simulink model "Simulink_asserv_Disc_10Avril_V2023a"  (R2023a)
settings: Solver=ode45  StartTime=0.0  StopTime=2500  FixedStep=0.01  RelTol=1e-3
undefined symbols (not defined in the file): AmbiantTemp, CondSig_mesureTemp_Gain, CondSig_mesureTemp_Vsub, Consigne1_Temps, Consigne1_Valeur, Consigne2_Temps, Consigne2_Valeur, Consigne3_Temps, Consigne3_Valeur, DivTen_mesureTemp_R_pullup, DivTen_mesureTemp_Vcc, Gain_Comparateur_VoltageControle, GuT1_Denominateur, GuT1_Numerateur, GuT2_Denominateur, GuT2_Numerateur, GuT3_Denominateur, GuT3_Numerateur, NbrsBits_ADC, NbrsBits_DAC, Perturbation_Resistance, Perturbation_TempsApplication, Perturbation_Tension, PerturbT1_Denominateur, PerturbT1_Numerateur, PerturbT2_Denominateur, PerturbT2_Numerateur, PerturbT3_Denominateur, PerturbT3_Numerateur, RC_deno, Regulateur_Denominateur, Regulateur_Numerateur, SaturationLimite_inferieure, SaturationLimite_superieure, setupDelay, SourceCourant_Gain_Vcontrole_vers_A, T1T3_Denominateur, T1T3_Numerateur, T2T3_Denominateur, T2T3_Numerateur, ThermoRes_SH_A, ThermoRes_SH_B, ThermoRes_SH_C, ThermoRes_SH_D, ThermoRes_SH_R_nom, ThermoRes_SHTEMP_A, ThermoRes_SHTEMP_B, ThermoRes_SHTEMP_C, ThermoRes_SHTEMP_D
libraries: simulink x2
settings Model: Creator=alcot161  LastModifiedBy=alcot161
settings RTWCC: GPUComputeCapability=5.0

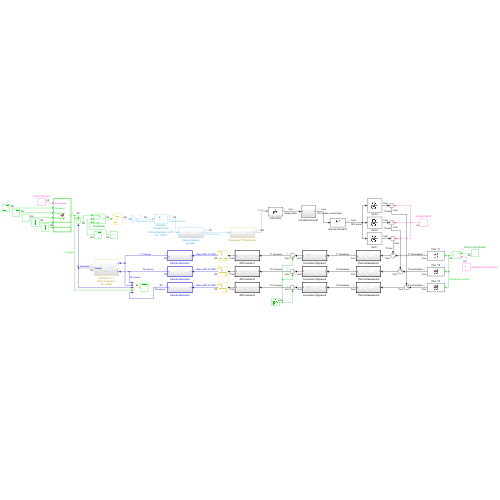
[thumbnail: Simulink's stored preview of the top-level diagram]
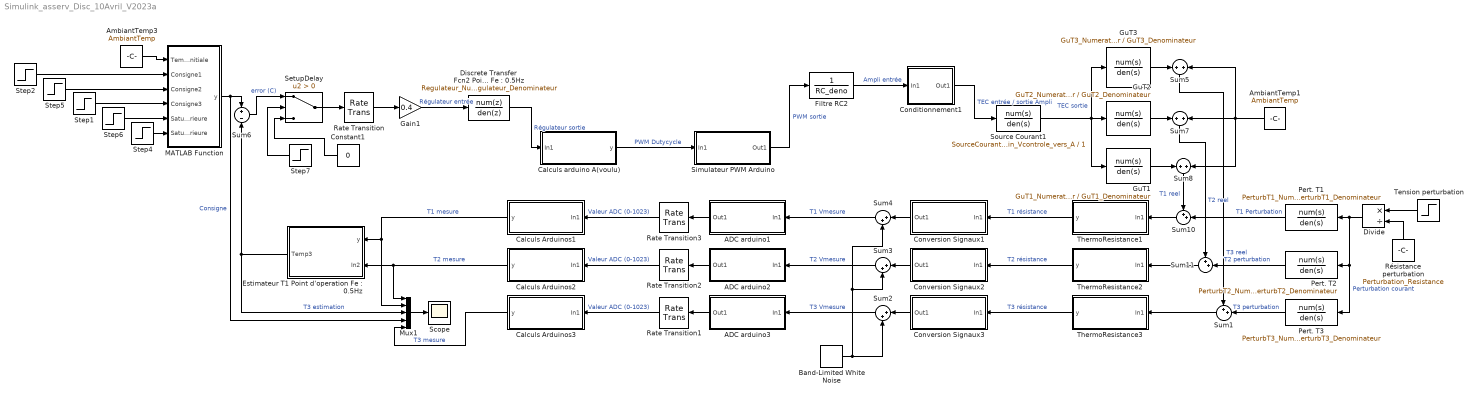
== system Simulink_asserv_Disc_10Avril_V2023a ==
  ADC arduino1 : Subsystem  TreatAsAtomicUnit=on
  ADC arduino2 : Subsystem  TreatAsAtomicUnit=on
  ADC arduino3 : Subsystem  TreatAsAtomicUnit=on
  AmbiantTemp1 : Constant  Value=AmbiantTemp
  AmbiantTemp3 : Constant  Value=AmbiantTemp
  Band-Limited White Noise : simulink/Sources/Band-Limited White Noise  Cov=BruitMesure  Ts=0.05  seed=[23341]
  Calculs Arduinos1 : Subsystem  TreatAsAtomicUnit=on
  Calculs Arduinos2 : Subsystem  TreatAsAtomicUnit=on
  Calculs Arduinos3 : Subsystem  TreatAsAtomicUnit=on
  "Calculs arduino A(voulu) " : Subsystem
  Conditionnement1 : Subsystem
  Constant1 : Constant  Value=0  SampleTime=0.05
  Conversion Signaux1 : Subsystem  TreatAsAtomicUnit=on
  Conversion Signaux2 : Subsystem  TreatAsAtomicUnit=on
  Conversion Signaux3 : Subsystem  TreatAsAtomicUnit=on
  "Discrete Transfer Fcn2 Point d'operation : 27C Fe : 0.5Hz" : DiscreteTransferFcn  Numerator=Regulateur_Numerateur  Denominator=Regulateur_Denominateur
  Divide : Product  Inputs=*/
  "Estimateur T1 Point d'operation Fe : 0.5Hz" : Subsystem
  Filtre RC2 : TransferFcn  Denominator=RC_deno
  Gain1 : Gain  Gain=0.4
  GuT1 : TransferFcn  Numerator=GuT1_Numerateur  Denominator=GuT1_Denominateur
  GuT2 : TransferFcn  Numerator=GuT2_Numerateur  Denominator=GuT2_Denominateur
  GuT3 : TransferFcn  Numerator=GuT3_Numerateur  Denominator=GuT3_Denominateur
  MATLAB Function : MATLAB Function  TreatAsAtomicUnit=on
  Mux1 : Mux  Inputs=5
  Pert. T1 : TransferFcn  Numerator=PerturbT1_Numerateur  Denominator=PerturbT1_Denominateur
  Pert. T2 : TransferFcn  Numerator=PerturbT2_Numerateur  Denominator=PerturbT2_Denominateur
  Pert. T3 : TransferFcn  Numerator=PerturbT3_Numerateur  Denominator=PerturbT3_Denominateur
  Rate Transition : RateTransition  OutPortSampleTime=PeriodEchant_asserv
  Rate Transition1 : RateTransition  OutPortSampleTime=PeriodeEchant_temp
  Rate Transition2 : RateTransition  OutPortSampleTime=PeriodeEchant_temp
  Rate Transition3 : RateTransition  OutPortSampleTime=PeriodeEchant_temp
  Résistance perturbation : Constant  Value=Perturbation_Resistance
  Scope : Scope
  SetupDelay : Switch  Criteria=u2 > Threshold  SaturateOnIntegerOverflow=off  InputSameDT=off
  Simulateur PWM Arduino : Subsystem
  Source Courant1 : TransferFcn  Numerator=SourceCourant_Gain_Vcontrole_vers_A  Denominator=1
  Step1 : Step  Time=Consigne3_Temps  After=Consigne3_Valeur  SampleTime=0.05
  Step2 : Step  Time=Consigne1_Temps  After=Consigne1_Valeur  SampleTime=0.05
  Step4 : Step  Time=0  After=SaturationLimite_inferieure  SampleTime=0.05
  Step5 : Step  Time=Consigne2_Temps  After=Consigne2_Valeur  SampleTime=0.05
  Step6 : Step  Time=0  After=SaturationLimite_superieure  SampleTime=0.05
  Step7 : Step  Time=setupDelay  SampleTime=0.05
  Sum1 : Sum  Inputs=++|
  Sum10 : Sum  Inputs=++|
  Sum11 : Sum  Inputs=++|
  Sum2 : Sum  Inputs=|++
  Sum3 : Sum  Inputs=|++
  Sum4 : Sum  Inputs=|++
  Sum5 : Sum  Inputs=+|+
  Sum6 : Sum  Inputs=+|-
  Sum7 : Sum  Inputs=+|+
  Sum8 : Sum  Inputs=+|+
  Tension perturbation : Step  Time=Perturbation_TempsApplication  After=Perturbation_Tension  SampleTime=0.05
  ThermoResistance1 : Subsystem  TreatAsAtomicUnit=on
  ThermoResistance2 : Subsystem  TreatAsAtomicUnit=on
  ThermoResistance3 : Subsystem  TreatAsAtomicUnit=on
  wires:
  ThermoResistance2/1(y) -> Conversion Signaux2/1(In1)  "T2 résistance"
  GuT2/1 -> Sum7/1
  Conversion Signaux2/1(Out1) -> Sum3/1
  Rate Transition2/1 -> Calculs Arduinos2/1(In1)  "Valeur ADC (0-1023)"
  Simulateur PWM Arduino/1(Out1) -> Filtre RC2/1  "PWM sortie"
  Step5/1 -> MATLAB Function/3(Consigne2)
  Conversion Signaux1/1(Out1) -> Sum4/1
  AmbiantTemp1/1 -> Sum5/2, Sum8/2, Sum7/2
  Filtre RC2/1 -> Conditionnement1/1(In1)  "Ampli entrée"
  Calculs Arduinos1/1(y) -> Mux1/2, "Estimateur T1 Point d'operation Fe : 0.5Hz"/1(y)  "T1 mesure"
  Rate Transition3/1 -> Calculs Arduinos1/1(In1)  "Valeur ADC (0-1023)"
  "Calculs arduino A(voulu) "/1(y) -> Simulateur PWM Arduino/1(In1)  "PWM Dutycycle"
  Calculs Arduinos2/1(y) -> "Estimateur T1 Point d'operation Fe : 0.5Hz"/2(In2), Mux1/1  "T2 mesure"
  Source Courant1/1 -> GuT3/1, GuT1/1, GuT2/1  "TEC sortie"
  ThermoResistance1/1(y) -> Conversion Signaux1/1(In1)  "T1 résistance"
  Sum7/1 -> Sum11/1  "T2 reel"
  Conditionnement1/1(Out1) -> Source Courant1/1  "TEC entrée / sortie Ampli"
  GuT1/1 -> Sum8/1
  GuT3/1 -> Sum5/1
  "Discrete Transfer Fcn2 Point d'operation : 27C Fe : 0.5Hz"/1 -> "Calculs arduino A(voulu) "/1(In1)  "Régulateur sortie"
  "Estimateur T1 Point d'operation Fe : 0.5Hz"/1(Temp3) -> Sum6/2, Mux1/3  "T3 estimation"
  Gain1/1 -> "Discrete Transfer Fcn2 Point d'operation : 27C Fe : 0.5Hz"/1  "Régulateur entrée"
  Sum6/1 -> SetupDelay/1  "error (C)"
  SetupDelay/1 -> Rate Transition/1
  Sum8/1 -> Sum10/1  "T1 reel"
  Sum10/1 -> ThermoResistance1/1(In1)
  Sum11/1 -> ThermoResistance2/1(In1)
  Step1/1 -> MATLAB Function/4(Consigne3)
  Résistance perturbation/1 -> Divide/2
  Tension perturbation/1 -> Divide/1
  Divide/1 -> Pert. T3/1, Pert. T2/1, Pert. T1/1  "Perturbation courant"
  Pert. T1/1 -> Sum10/2  "T1 Perturbation"
  AmbiantTemp3/1 -> MATLAB Function/1(TempInitiale)
  Step2/1 -> MATLAB Function/2(Consigne1)
  MATLAB Function/1(y) -> Mux1/4, Sum6/1  "Consigne"
  Calculs Arduinos3/1(y) -> Mux1/5  "T3 mesure"
  ThermoResistance3/1(y) -> Conversion Signaux3/1(In1)  "T3 résistance"
  Rate Transition1/1 -> Calculs Arduinos3/1(In1)  "Valeur ADC (0-1023)"
  Conversion Signaux3/1(Out1) -> Sum2/1
  Sum5/1 -> Sum1/1  "T3 reel"
  Pert. T2/1 -> Sum11/2  "T2 perturbation"
  Pert. T3/1 -> Sum1/2  "T3 perturbation"
  Sum1/1 -> ThermoResistance3/1(In1)
  Step4/1 -> MATLAB Function/6(SaturationLimiteInferieure)
  Step6/1 -> MATLAB Function/5(SaturationLimiteSuperieure)
  Constant1/1 -> SetupDelay/3
  Step7/1 -> SetupDelay/2
  Mux1/1 -> Scope/1
  Sum2/1 -> ADC arduino3/1(In1)  "T3 Vmesure"
  Sum3/1 -> ADC arduino2/1(In1)  "T2 Vmesure"
  Sum4/1 -> ADC arduino1/1(In1)  "T1 Vmesure"
  Band-Limited White Noise/1 -> Sum2/2, Sum4/2, Sum3/2
  ADC arduino3/1(Out1) -> Rate Transition1/1
  ADC arduino1/1(Out1) -> Rate Transition3/1
  ADC arduino2/1(Out1) -> Rate Transition2/1
  Rate Transition/1 -> Gain1/1

== system Simulink_asserv_Disc_10Avril_V2023a/ADC arduino1 ==
  In1 : Inport
  Floor : Rounding
  Gain2 : Gain  Gain=2^NbrsBits_ADC/5
  Out1 : Outport
  wires:
  In1/1 -> Gain2/1
  Gain2/1 -> Floor/1
  Floor/1 -> Out1/1

== system Simulink_asserv_Disc_10Avril_V2023a/ADC arduino2 ==
  In1 : Inport
  Floor : Rounding
  Gain2 : Gain  Gain=2^NbrsBits_ADC/5
  Out1 : Outport
  wires:
  Floor/1 -> Out1/1
  In1/1 -> Gain2/1
  Gain2/1 -> Floor/1

== system Simulink_asserv_Disc_10Avril_V2023a/ADC arduino3 ==
  In1 : Inport
  Floor : Rounding
  Gain2 : Gain  Gain=2^NbrsBits_ADC/5
  Out1 : Outport
  wires:
  Floor/1 -> Out1/1
  In1/1 -> Gain2/1
  Gain2/1 -> Floor/1

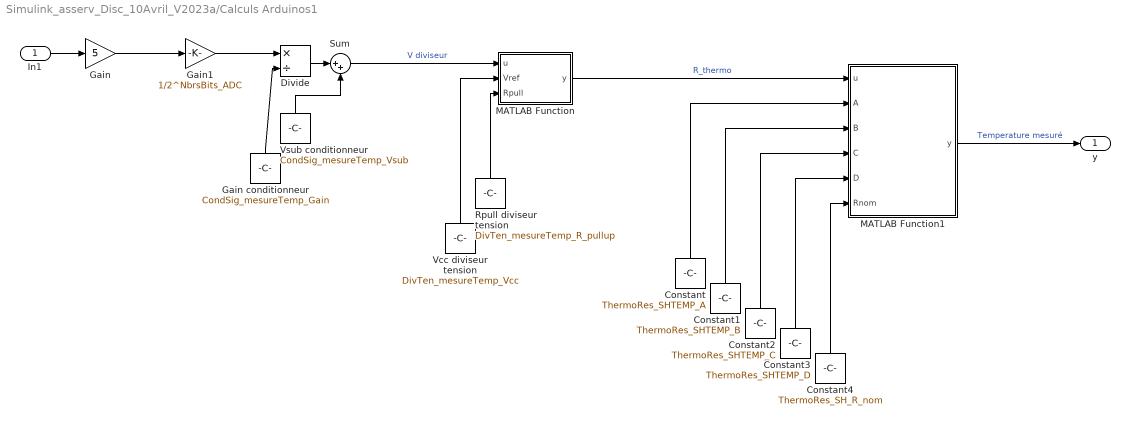
== system Simulink_asserv_Disc_10Avril_V2023a/Calculs Arduinos1 ==
  In1 : Inport
  Constant : Constant  Value=ThermoRes_SHTEMP_A
  Constant1 : Constant  Value=ThermoRes_SHTEMP_B
  Constant2 : Constant  Value=ThermoRes_SHTEMP_C
  Constant3 : Constant  Value=ThermoRes_SHTEMP_D
  Constant4 : Constant  Value=ThermoRes_SH_R_nom
  Divide : Product  Inputs=*/
  Gain : Gain  Gain=5
  Gain conditionneur : Constant  Value=CondSig_mesureTemp_Gain
  Gain1 : Gain  Gain=1/2^NbrsBits_ADC
  MATLAB Function : MATLAB Function  TreatAsAtomicUnit=on
  MATLAB Function1 : MATLAB Function  TreatAsAtomicUnit=on
  Rpull diviseur tension : Constant  Value=DivTen_mesureTemp_R_pullup
  Sum : Sum  Inputs=|++
  Vcc diviseur tension : Constant  Value=DivTen_mesureTemp_Vcc
  Vsub conditionneur : Constant  Value=CondSig_mesureTemp_Vsub
  y : Outport
  wires:
  In1/1 -> Gain/1
  Gain/1 -> Gain1/1
  Gain conditionneur/1 -> Divide/2
  Divide/1 -> Sum/1
  Vsub conditionneur/1 -> Sum/2
  Sum/1 -> MATLAB Function/1(u)  "V diviseur"
  Rpull diviseur tension/1 -> MATLAB Function/3(Rpull)
  Vcc diviseur tension/1 -> MATLAB Function/2(Vref)
  MATLAB Function/1(y) -> MATLAB Function1/1(u)  "R_thermo"
  Constant/1 -> MATLAB Function1/2(A)
  Constant1/1 -> MATLAB Function1/3(B)
  Constant2/1 -> MATLAB Function1/4(C)
  Constant3/1 -> MATLAB Function1/5(D)
  Constant4/1 -> MATLAB Function1/6(Rnom)
  MATLAB Function1/1(y) -> y/1  "Temperature mesuré"
  Gain1/1 -> Divide/1

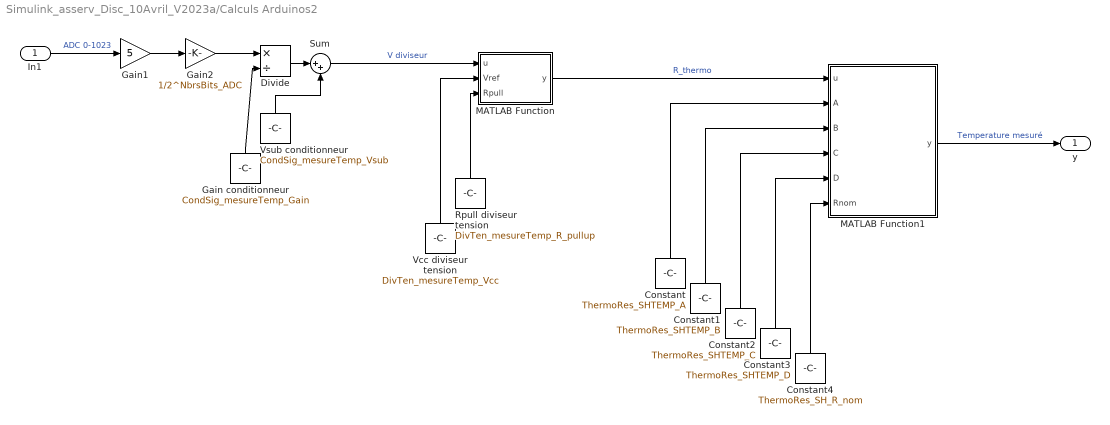
== system Simulink_asserv_Disc_10Avril_V2023a/Calculs Arduinos2 ==
  In1 : Inport
  Constant : Constant  Value=ThermoRes_SHTEMP_A
  Constant1 : Constant  Value=ThermoRes_SHTEMP_B
  Constant2 : Constant  Value=ThermoRes_SHTEMP_C
  Constant3 : Constant  Value=ThermoRes_SHTEMP_D
  Constant4 : Constant  Value=ThermoRes_SH_R_nom
  Divide : Product  Inputs=*/
  Gain conditionneur : Constant  Value=CondSig_mesureTemp_Gain
  Gain1 : Gain  Gain=5
  Gain2 : Gain  Gain=1/2^NbrsBits_ADC
  MATLAB Function : MATLAB Function  TreatAsAtomicUnit=on
  MATLAB Function1 : MATLAB Function  TreatAsAtomicUnit=on
  Rpull diviseur tension : Constant  Value=DivTen_mesureTemp_R_pullup
  Sum : Sum  Inputs=|++
  Vcc diviseur tension : Constant  Value=DivTen_mesureTemp_Vcc
  Vsub conditionneur : Constant  Value=CondSig_mesureTemp_Vsub
  y : Outport
  wires:
  Gain conditionneur/1 -> Divide/2
  Divide/1 -> Sum/1
  Vsub conditionneur/1 -> Sum/2
  Sum/1 -> MATLAB Function/1(u)  "V diviseur"
  Rpull diviseur tension/1 -> MATLAB Function/3(Rpull)
  Vcc diviseur tension/1 -> MATLAB Function/2(Vref)
  MATLAB Function/1(y) -> MATLAB Function1/1(u)  "R_thermo"
  Constant/1 -> MATLAB Function1/2(A)
  Constant1/1 -> MATLAB Function1/3(B)
  Constant2/1 -> MATLAB Function1/4(C)
  Constant3/1 -> MATLAB Function1/5(D)
  Constant4/1 -> MATLAB Function1/6(Rnom)
  MATLAB Function1/1(y) -> y/1  "Temperature mesuré"
  Gain2/1 -> Divide/1
  In1/1 -> Gain1/1  "ADC 0-1023"
  Gain1/1 -> Gain2/1

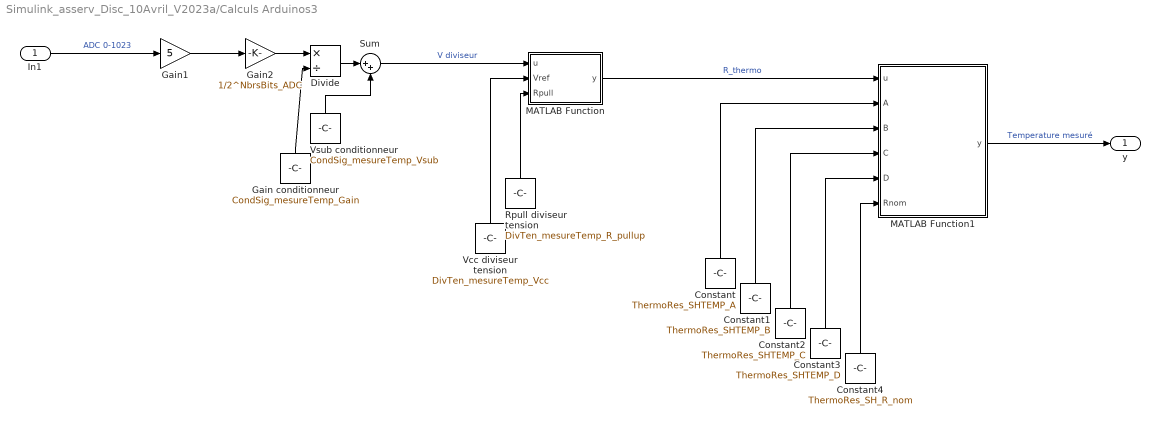
== system Simulink_asserv_Disc_10Avril_V2023a/Calculs Arduinos3 ==
  In1 : Inport
  Constant : Constant  Value=ThermoRes_SHTEMP_A
  Constant1 : Constant  Value=ThermoRes_SHTEMP_B
  Constant2 : Constant  Value=ThermoRes_SHTEMP_C
  Constant3 : Constant  Value=ThermoRes_SHTEMP_D
  Constant4 : Constant  Value=ThermoRes_SH_R_nom
  Divide : Product  Inputs=*/
  Gain conditionneur : Constant  Value=CondSig_mesureTemp_Gain
  Gain1 : Gain  Gain=5
  Gain2 : Gain  Gain=1/2^NbrsBits_ADC
  MATLAB Function : MATLAB Function  TreatAsAtomicUnit=on
  MATLAB Function1 : MATLAB Function  TreatAsAtomicUnit=on
  Rpull diviseur tension : Constant  Value=DivTen_mesureTemp_R_pullup
  Sum : Sum  Inputs=|++
  Vcc diviseur tension : Constant  Value=DivTen_mesureTemp_Vcc
  Vsub conditionneur : Constant  Value=CondSig_mesureTemp_Vsub
  y : Outport
  wires:
  Gain conditionneur/1 -> Divide/2
  Divide/1 -> Sum/1
  Vsub conditionneur/1 -> Sum/2
  Sum/1 -> MATLAB Function/1(u)  "V diviseur"
  Rpull diviseur tension/1 -> MATLAB Function/3(Rpull)
  Vcc diviseur tension/1 -> MATLAB Function/2(Vref)
  MATLAB Function/1(y) -> MATLAB Function1/1(u)  "R_thermo"
  Constant/1 -> MATLAB Function1/2(A)
  Constant1/1 -> MATLAB Function1/3(B)
  Constant2/1 -> MATLAB Function1/4(C)
  Constant3/1 -> MATLAB Function1/5(D)
  Constant4/1 -> MATLAB Function1/6(Rnom)
  MATLAB Function1/1(y) -> y/1  "Temperature mesuré"
  In1/1 -> Gain1/1  "ADC 0-1023"
  Gain2/1 -> Divide/1
  Gain1/1 -> Gain2/1

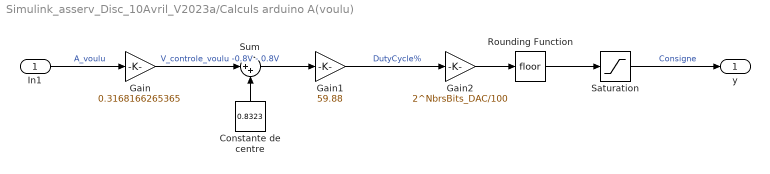
== system Simulink_asserv_Disc_10Avril_V2023a/Calculs arduino A(voulu)  ==
  In1 : Inport
  Constante de centre : Constant  Value=0.8323
  Gain : Gain  Gain=0.3168166265365
  Gain1 : Gain  Gain=59.88
  Gain2 : Gain  Gain=2^NbrsBits_DAC/100
  Rounding Function : Rounding
  Saturation : Saturate  UpperLimit=2^NbrsBits_DAC-1  LowerLimit=0
  Sum : Sum  Inputs=|++
  y : Outport
  wires:
  In1/1 -> Gain/1  "A_voulu"
  Gain/1 -> Sum/1  "V_controle_voulu -0.8V - 0.8V"
  Sum/1 -> Gain1/1
  Constante de centre/1 -> Sum/2
  Gain1/1 -> Gain2/1  "DutyCycle%"
  Gain2/1 -> Rounding Function/1
  Rounding Function/1 -> Saturation/1
  Saturation/1 -> y/1  "Consigne"

== system Simulink_asserv_Disc_10Avril_V2023a/Conditionnement1 ==
  In1 : Inport
  Constant : Constant  Value=2.5
  Gain : Gain  Gain=Gain_Comparateur_VoltageControle
  Subtract : Sum  Inputs=+-
  Out1 : Outport
  wires:
  In1/1 -> Subtract/1
  Constant/1 -> Subtract/2
  Subtract/1 -> Gain/1
  Gain/1 -> Out1/1

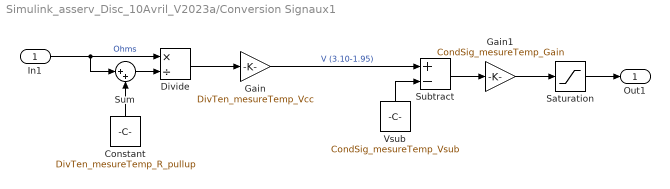
== system Simulink_asserv_Disc_10Avril_V2023a/Conversion Signaux1 ==
  In1 : Inport
  Constant : Constant  Value=DivTen_mesureTemp_R_pullup
  Divide : Product  Inputs=*/
  Gain : Gain  Gain=DivTen_mesureTemp_Vcc
  Gain1 : Gain  Gain=CondSig_mesureTemp_Gain
  Saturation : Saturate  UpperLimit=5  LowerLimit=0
  Subtract : Sum  Inputs=+-
  Sum : Sum  Inputs=|++
  Vsub : Constant  Value=CondSig_mesureTemp_Vsub
  Out1 : Outport
  wires:
  In1/1 -> Sum/1, Divide/1  "Ohms"
  Sum/1 -> Divide/2
  Constant/1 -> Sum/2
  Divide/1 -> Gain/1
  Vsub/1 -> Subtract/2
  Subtract/1 -> Gain1/1
  Gain1/1 -> Saturation/1
  Saturation/1 -> Out1/1
  Gain/1 -> Subtract/1  "V (3.10-1.95)"

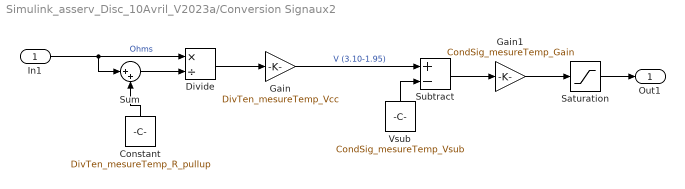
== system Simulink_asserv_Disc_10Avril_V2023a/Conversion Signaux2 ==
  In1 : Inport
  Constant : Constant  Value=DivTen_mesureTemp_R_pullup
  Divide : Product  Inputs=*/
  Gain : Gain  Gain=DivTen_mesureTemp_Vcc
  Gain1 : Gain  Gain=CondSig_mesureTemp_Gain
  Saturation : Saturate  UpperLimit=5  LowerLimit=0
  Subtract : Sum  Inputs=+-
  Sum : Sum  Inputs=|++
  Vsub : Constant  Value=CondSig_mesureTemp_Vsub
  Out1 : Outport
  wires:
  In1/1 -> Sum/1, Divide/1  "Ohms"
  Sum/1 -> Divide/2
  Constant/1 -> Sum/2
  Divide/1 -> Gain/1
  Vsub/1 -> Subtract/2
  Subtract/1 -> Gain1/1
  Gain1/1 -> Saturation/1
  Saturation/1 -> Out1/1
  Gain/1 -> Subtract/1  "V (3.10-1.95)"

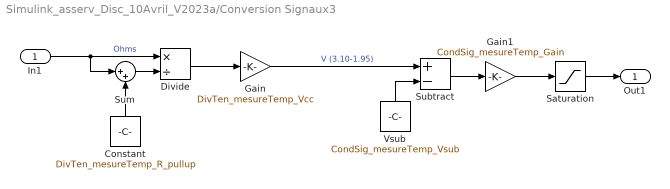
== system Simulink_asserv_Disc_10Avril_V2023a/Conversion Signaux3 ==
  In1 : Inport
  Constant : Constant  Value=DivTen_mesureTemp_R_pullup
  Divide : Product  Inputs=*/
  Gain : Gain  Gain=DivTen_mesureTemp_Vcc
  Gain1 : Gain  Gain=CondSig_mesureTemp_Gain
  Saturation : Saturate  UpperLimit=5  LowerLimit=0
  Subtract : Sum  Inputs=+-
  Sum : Sum  Inputs=|++
  Vsub : Constant  Value=CondSig_mesureTemp_Vsub
  Out1 : Outport
  wires:
  In1/1 -> Sum/1, Divide/1  "Ohms"
  Sum/1 -> Divide/2
  Constant/1 -> Sum/2
  Divide/1 -> Gain/1
  Vsub/1 -> Subtract/2
  Subtract/1 -> Gain1/1
  Gain1/1 -> Saturation/1
  Saturation/1 -> Out1/1
  Gain/1 -> Subtract/1  "V (3.10-1.95)"

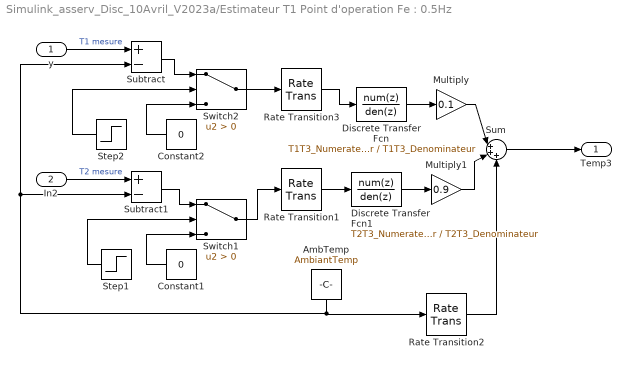
== system Simulink_asserv_Disc_10Avril_V2023a/Estimateur T1 Point d'operation Fe : 0.5Hz ==
  y : Inport
  In2 : Inport  Port=2
  AmbTemp : Constant  Value=AmbiantTemp  SampleTime=0.05
  Constant1 : Constant  Value=0  SampleTime=0.05
  Constant2 : Constant  Value=0  SampleTime=0.05
  Discrete Transfer Fcn : DiscreteTransferFcn  Numerator=T1T3_Numerateur  Denominator=T1T3_Denominateur
  Discrete Transfer Fcn1 : DiscreteTransferFcn  Numerator=T2T3_Numerateur  Denominator=T2T3_Denominateur
  Multiply : Gain  Gain=0.1
  Multiply1 : Gain  Gain=0.9
  Rate Transition1 : RateTransition  OutPortSampleTime=PeriodeEchant_temp
  Rate Transition2 : RateTransition  OutPortSampleTime=PeriodeEchant_temp
  Rate Transition3 : RateTransition  OutPortSampleTime=PeriodeEchant_temp
  Step1 : Step  Time=setupDelay  SampleTime=0.05
  Step2 : Step  Time=setupDelay  SampleTime=0.05
  Subtract : Sum  Inputs=+-
  Subtract1 : Sum  Inputs=+-
  Sum : Sum  Inputs=|+++
  Switch1 : Switch  Criteria=u2 > Threshold  SaturateOnIntegerOverflow=off  InputSameDT=off
  Switch2 : Switch  Criteria=u2 > Threshold  SaturateOnIntegerOverflow=off  InputSameDT=off
  Temp3 : Outport
  wires:
  In2/1 -> Subtract1/1  "T2 mesure"
  Multiply/1 -> Sum/1
  Multiply1/1 -> Sum/2
  y/1 -> Subtract/1  "T1 mesure"
  Sum/1 -> Temp3/1
  Discrete Transfer Fcn/1 -> Multiply/1
  Discrete Transfer Fcn1/1 -> Multiply1/1
  AmbTemp/1 -> Subtract/2, Subtract1/2, Rate Transition2/1
  Constant2/1 -> Switch2/3
  Step2/1 -> Switch2/2
  Subtract/1 -> Switch2/1
  Switch2/1 -> Rate Transition3/1
  Subtract1/1 -> Switch1/1
  Switch1/1 -> Rate Transition1/1
  Step1/1 -> Switch1/2
  Constant1/1 -> Switch1/3
  Rate Transition3/1 -> Discrete Transfer Fcn/1
  Rate Transition1/1 -> Discrete Transfer Fcn1/1
  Rate Transition2/1 -> Sum/3

== system Simulink_asserv_Disc_10Avril_V2023a/Simulateur PWM Arduino ==
  In1 : Inport
  Gain1 : Gain  Gain=1/((2^NbrsBits_DAC)-1)
  Gain2 : Gain  Gain=5
  PWM : simulink/Discontinuities/PWM  DisableCoverage=on  Period=0.00204  InitialDelay=0  DisallowZeroDutyCycle=off  RunAtFixedTimeIntervals=off  SampleTime=0.1
  Out1 : Outport
  wires:
  PWM/1 -> Gain2/1  "PWM / DAC sortie"
  Gain2/1 -> Out1/1
  In1/1 -> Gain1/1  "DutyCycle%"
  Gain1/1 -> PWM/1

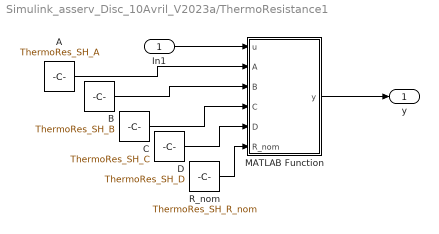
== system Simulink_asserv_Disc_10Avril_V2023a/ThermoResistance1 ==
  In1 : Inport
  A : Constant  Value=ThermoRes_SH_A
  B : Constant  Value=ThermoRes_SH_B
  C : Constant  Value=ThermoRes_SH_C
  D : Constant  Value=ThermoRes_SH_D
  MATLAB Function : MATLAB Function  TreatAsAtomicUnit=on
  R_nom : Constant  Value=ThermoRes_SH_R_nom
  y : Outport
  wires:
  In1/1 -> MATLAB Function/1(u)
  MATLAB Function/1(y) -> y/1
  A/1 -> MATLAB Function/2(A)
  B/1 -> MATLAB Function/3(B)
  C/1 -> MATLAB Function/4(C)
  D/1 -> MATLAB Function/5(D)
  R_nom/1 -> MATLAB Function/6(R_nom)

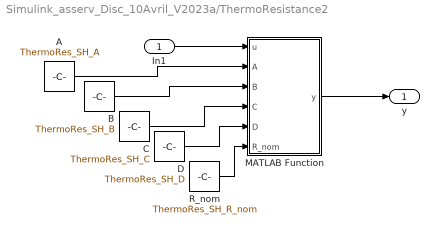
== system Simulink_asserv_Disc_10Avril_V2023a/ThermoResistance2 ==
  In1 : Inport
  A : Constant  Value=ThermoRes_SH_A
  B : Constant  Value=ThermoRes_SH_B
  C : Constant  Value=ThermoRes_SH_C
  D : Constant  Value=ThermoRes_SH_D
  MATLAB Function : MATLAB Function  TreatAsAtomicUnit=on
  R_nom : Constant  Value=ThermoRes_SH_R_nom
  y : Outport
  wires:
  In1/1 -> MATLAB Function/1(u)
  MATLAB Function/1(y) -> y/1
  A/1 -> MATLAB Function/2(A)
  B/1 -> MATLAB Function/3(B)
  C/1 -> MATLAB Function/4(C)
  D/1 -> MATLAB Function/5(D)
  R_nom/1 -> MATLAB Function/6(R_nom)

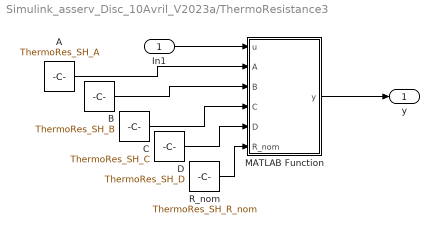
== system Simulink_asserv_Disc_10Avril_V2023a/ThermoResistance3 ==
  In1 : Inport
  A : Constant  Value=ThermoRes_SH_A
  B : Constant  Value=ThermoRes_SH_B
  C : Constant  Value=ThermoRes_SH_C
  D : Constant  Value=ThermoRes_SH_D
  MATLAB Function : MATLAB Function  TreatAsAtomicUnit=on
  R_nom : Constant  Value=ThermoRes_SH_R_nom
  y : Outport
  wires:
  In1/1 -> MATLAB Function/1(u)
  MATLAB Function/1(y) -> y/1
  A/1 -> MATLAB Function/2(A)
  B/1 -> MATLAB Function/3(B)
  C/1 -> MATLAB Function/4(C)
  D/1 -> MATLAB Function/5(D)
  R_nom/1 -> MATLAB Function/6(R_nom)

== matlab function Simulink_asserv_Disc_10Avril_V2023a/ThermoResistance1/MATLAB Function ==
  data: u input; y output; A input; B input; C input; D input; R_nom input
function y = fcn(u, A, B, C, D, R_nom)
   
y = R_nom * exp(A + (B/(u+273.15)) + (C/((u + 273.15)^2)) + (D/((u + 273.15)^3)));

== matlab function Simulink_asserv_Disc_10Avril_V2023a/ThermoResistance2/MATLAB Function ==
  data: u input; y output; A input; B input; C input; D input; R_nom input
function y = fcn(u, A, B, C, D, R_nom)
   
y = R_nom * exp(A + (B/(u+273.15)) + (C/((u + 273.15)^2)) + (D/((u + 273.15)^3)));

== matlab function Simulink_asserv_Disc_10Avril_V2023a/MATLAB Function ==
  data: TempInitiale input; y output; Consigne1 input; Consigne2 input; Consigne3 input; SaturationLimiteSuperieure input; SaturationLimiteInferieure input
function y = fcn(TempInitiale, Consigne1, Consigne2, Consigne3, SaturationLimiteSuperieure, SaturationLimiteInferieure)
   
y = TempInitiale;
if (Consigne1 ~= 0)
    y = Consigne1;
end
if (Consigne2 ~= 0)
    y = Consigne2;
end
if (Consigne3 ~= 0)
    y = Consigne3;
end
if (y > SaturationLimiteSuperieure)
    y = SaturationLimiteSuperieure;
end
if (y < SaturationLimiteInferieure)
    y = SaturationLimiteInferieure;
end

== matlab function Simulink_asserv_Disc_10Avril_V2023a/Calculs Arduinos3/MATLAB Function ==
  data: u input; y output; Vref input; Rpull input
function y = fcn(u, Vref, Rpull)

y = Rpull * (u/(Vref-u));

== matlab function Simulink_asserv_Disc_10Avril_V2023a/Calculs Arduinos3/MATLAB Function1 ==
  data: u input; y output; A input; B input; C input; D input; Rnom input
function y = fcn(u, A, B, C, D, Rnom)
    invT = A + B*log(u/Rnom) + C*(log(u/Rnom))^2 + D*(log(u/Rnom))^3;
    T = (1/invT) - 273.15;
y = T;

== matlab function Simulink_asserv_Disc_10Avril_V2023a/ThermoResistance3/MATLAB Function ==
  data: u input; y output; A input; B input; C input; D input; R_nom input
function y = fcn(u, A, B, C, D, R_nom)
   
y = R_nom * exp(A + (B/(u+273.15)) + (C/((u + 273.15)^2)) + (D/((u + 273.15)^3)));

== matlab function Simulink_asserv_Disc_10Avril_V2023a/Calculs Arduinos1/MATLAB Function ==
  data: u input; y output; Vref input; Rpull input
function y = fcn(u, Vref, Rpull)

y = Rpull * (u/(Vref-u));

== matlab function Simulink_asserv_Disc_10Avril_V2023a/Calculs Arduinos1/MATLAB Function1 ==
  data: u input; y output; A input; B input; C input; D input; Rnom input
function y = fcn(u, A, B, C, D, Rnom)
    invT = A + B*log(u/Rnom) + C*(log(u/Rnom))^2 + D*(log(u/Rnom))^3;
    T = (1/invT) - 273.15;
y = T;

== matlab function Simulink_asserv_Disc_10Avril_V2023a/Calculs Arduinos2/MATLAB Function ==
  data: u input; y output; Vref input; Rpull input
function y = fcn(u, Vref, Rpull)

y = Rpull * (u/(Vref-u));

== matlab function Simulink_asserv_Disc_10Avril_V2023a/Calculs Arduinos2/MATLAB Function1 ==
  data: u input; y output; A input; B input; C input; D input; Rnom input
function y = fcn(u, A, B, C, D, Rnom)
    invT = A + B*log(u/Rnom) + C*(log(u/Rnom))^2 + D*(log(u/Rnom))^3;
    T = (1/invT) - 273.15;
y = T;
